simulink model "Echo_and_Reverberation"  (R2018a)
settings: Solver=VariableStepDiscrete  StartTime=0.0  StopTime=10.0  RelTol=1e-3
libraries: dspvision x4
settings Model: Creator=ashwin  LastModifiedBy=ashwin

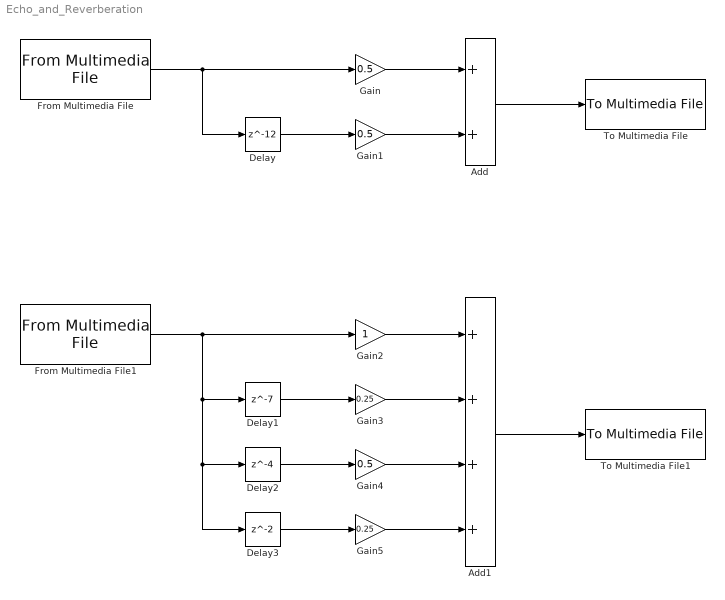
== system Echo_and_Reverberation ==
  Add : Sum
  Add1 : Sum  Inputs=++++
  Delay : Delay  DelayLength=12
  Delay1 : Delay  DelayLength=7
  Delay2 : Delay  DelayLength=4
  Delay3 : Delay
  From Multimedia File : dspvision/From Multimedia File  inputFilename=/Users/ashwin/Downloads/IET MATLAB:Simulink Course/Models/Signal_Processing/speech_dft.wav  loop=on  numPlays=inf  outputStreams=Audio only  videoDataType=single  audioDataType=double  inheritSampleTime=on  userDefinedSampleTime=1/30  noAudioOutput=off  isIntensityVideo=off  fourcc=RGB  colorVideoFormat=Separate color signals  outputEOF=off  dataOrg=Column-major  audioFrameSize=1024  computeAudioFrameSize=off  outSamplingMode=Sample based
      settings: SourceProductBaseCode=VP
  From Multimedia File1 : dspvision/From Multimedia File  inputFilename=/Users/ashwin/Downloads/IET MATLAB:Simulink Course/Models/Signal_Processing/speech_dft.wav  loop=on  numPlays=inf  outputStreams=Audio only  videoDataType=single  audioDataType=double  inheritSampleTime=on  userDefinedSampleTime=1/30  noAudioOutput=off  isIntensityVideo=off  fourcc=RGB  colorVideoFormat=Separate color signals  outputEOF=off  dataOrg=Column-major  audioFrameSize=1024  computeAudioFrameSize=off  outSamplingMode=Sample based
      settings: SourceProductBaseCode=VP
  Gain : Gain  Gain=0.5
  Gain1 : Gain  Gain=0.5
  Gain2 : Gain
  Gain3 : Gain  Gain=0.25
  Gain4 : Gain  Gain=0.5
  Gain5 : Gain  Gain=0.25
  To Multimedia File : dspvision/To Multimedia File  outputFilename=/Users/ashwin/Downloads/IET MATLAB:Simulink Course/MATLAB_Code_Examples/echo.wav  streamSelection=Audio only  videoCompressor=None (uncompressed)  audioCompressor=None (uncompressed)  imagePorts=Separate color signals  fileType=WAV  audioDatatype=16-bit integer  fourcc=RGB  videoQuality=75  mj2000CompFactor=10
      settings: SourceProductName=Computer Vision System Toolbox  SourceProductBaseCode=VP
  To Multimedia File1 : dspvision/To Multimedia File  outputFilename=/Users/ashwin/Downloads/IET MATLAB:Simulink Course/MATLAB_Code_Examples/reverberation.wav  streamSelection=Audio only  videoCompressor=None (uncompressed)  audioCompressor=None (uncompressed)  imagePorts=Separate color signals  fileType=WAV  audioDatatype=16-bit integer  fourcc=RGB  videoQuality=75  mj2000CompFactor=10
      settings: SourceProductName=Computer Vision System Toolbox  SourceProductBaseCode=VP
  wires:
  From Multimedia File/1 -> Delay/1, Gain/1
  Delay/1 -> Gain1/1
  Gain/1 -> Add/1
  Gain1/1 -> Add/2
  Add/1 -> To Multimedia File/1
  Add1/1 -> To Multimedia File1/1
  Gain2/1 -> Add1/1
  From Multimedia File1/1 -> Delay3/1, Delay2/1, Delay1/1, Gain2/1
  Delay1/1 -> Gain3/1
  Delay2/1 -> Gain4/1
  Delay3/1 -> Gain5/1
  Gain4/1 -> Add1/3
  Gain3/1 -> Add1/2
  Gain5/1 -> Add1/4
